simulink model "AXI_QPSK_Tx"  (R2023b)
settings: Solver=FixedStepAuto  StartTime=0.0  StopTime=10/Rb  RelTol=1e-3
PreLoadFcn:
  | Rb = 1000;   % 1kbit / s
  | Rsym = Rb/2;   % 2 bits per symbol
  | Rsymbol = Rb/2;
  | OSR = 32;
  | f_error = 120;
  | 
  | design_filters_tx
values from neighbouring files (symbols this model uses):
  CIC_fine_Tx = 2^-(CIC_right_shift - CIC_left_shift - CIC_shift_Tx)    [design_filters_tx.m]
  fCIC = fCICcomp * R_CIC    (= 25600000)    [design_filters_tx.m]
  fHB = fRRC * R_HB    (= 4000)    [design_filters_tx.m]
  R_CICcomp = 2    [design_filters_tx.m]
  R_HB = 2    [design_filters_tx.m]
  R_RRC = 4    [design_filters_tx.m]
undefined symbols (not defined in the file or in its folder): AXI4, Lite
libraries: hdlBasic x309, hdlDSPIP x8, hdlsllib x2, vmcUtilities x1
(part 2 of 4)

== system AXI_QPSK_Tx/AXI_QPSK_Generator/M_AXIS_FFT ==
  tdata_in : Inport
  tvalid_in : Inport  Port=2
  tlast_in : Inport  Port=3
  tready_in : Inport  Port=4
  m_fft_axis_tdata : hdlBasic/Gateway Out  inherit_from_input=on  hdl_port=on  rows=1  columns=1  UseAsDAC=off  DACChannel='1'  interface=None  automatic_assignment=on  address_offset=hex2dec('00')  intf_name=''  intf_description=''  timing_constraint=None  locs_specified=off  LOCs={}  io_standard={}  XmcBlockStatus=1  maskContainerNames=group4  block_type=gatewayout  block_config=sysgen:gateway_out_config  block_width_w=590  block_height_w=620  block_width=620  block_height=750
  m_fft_axis_tlast : hdlBasic/Gateway Out  inherit_from_input=off  hdl_port=on  rows=1  columns=1  UseAsDAC=off  DACChannel='1'  interface=None  automatic_assignment=on  address_offset=hex2dec('00')  intf_name=''  intf_description=''  timing_constraint=None  locs_specified=off  LOCs={}  io_standard={}  XmcBlockStatus=1  maskContainerNames=group4  block_type=gatewayout  block_config=sysgen:gateway_out_config  block_width_w=590  block_height_w=620  block_width=620  block_height=750
  m_fft_axis_tready : hdlBasic/Gateway In  gui_display_data_type=Boolean  arith_type=Boolean  n_bits=16  bin_pt=14  preci_type=Single  exp_width=8  frac_width=24  rows=1  columns=1  quantization="Round  (unbiased: +/- Inf)"  overflow=Saturate  period=1/(fCIC)  UseAsADC=off  ADCChannel='1'  interface=None  automatic_assignment=on  address_offset=hex2dec('00')  intf_name=''  intf_description=''  default_value=0  timing_constraint=None  locs_specified=off  LOCs={}  io_standard={}  inherit_from_input=off  hdl_port=on  XmcBlockStatus=1  maskContainerNames=group4  block_type=gatewayin  block_config=sysgen:gateway_in_config  block_width_w=590  block_height_w=620  block_width=640  block_height=850
  m_fft_axis_tvalid : hdlBasic/Gateway Out  inherit_from_input=off  hdl_port=on  rows=1  columns=1  UseAsDAC=off  DACChannel='1'  interface=None  automatic_assignment=on  address_offset=hex2dec('00')  intf_name=''  intf_description=''  timing_constraint=None  locs_specified=off  LOCs={}  io_standard={}  XmcBlockStatus=1  maskContainerNames=group4  block_type=gatewayout  block_config=sysgen:gateway_out_config  block_width_w=590  block_height_w=620  block_width=620  block_height=750
  tdata_out : Outport  VectorParamsAs1DForOutWhenUnconnected=off
  tvalid_out : Outport  Port=2  VectorParamsAs1DForOutWhenUnconnected=off
  tlast_out : Outport  Port=3  VectorParamsAs1DForOutWhenUnconnected=off
  tready_out : Outport  Port=4  VectorParamsAs1DForOutWhenUnconnected=off
  wires:
  tready_in/1 -> m_fft_axis_tready/1
  m_fft_axis_tdata/1 -> tdata_out/1
  tdata_in/1 -> m_fft_axis_tdata/1
  m_fft_axis_tvalid/1 -> tvalid_out/1
  tvalid_in/1 -> m_fft_axis_tvalid/1
  m_fft_axis_tready/1 -> tready_out/1
  m_fft_axis_tlast/1 -> tlast_out/1
  tlast_in/1 -> m_fft_axis_tlast/1

== system AXI_QPSK_Tx/AXI_QPSK_Generator/M_AXIS_SYMBOL ==
  tdata_in : Inport
  tvalid_in : Inport  Port=2
  tlast_in : Inport  Port=3
  tready_in : Inport  Port=4
  m_symbol_axis_tdata : hdlBasic/Gateway Out  inherit_from_input=on  hdl_port=on  rows=1  columns=1  UseAsDAC=off  DACChannel='1'  interface=None  automatic_assignment=on  address_offset=hex2dec('00')  intf_name=''  intf_description=''  timing_constraint=None  locs_specified=off  LOCs={}  io_standard={}  XmcBlockStatus=1  maskContainerNames=group4  block_type=gatewayout  block_config=sysgen:gateway_out_config  block_width_w=590  block_height_w=620  block_width=620  block_height=750
  m_symbol_axis_tlast : hdlBasic/Gateway Out  inherit_from_input=off  hdl_port=on  rows=1  columns=1  UseAsDAC=off  DACChannel='1'  interface=None  automatic_assignment=on  address_offset=hex2dec('00')  intf_name=''  intf_description=''  timing_constraint=None  locs_specified=off  LOCs={}  io_standard={}  XmcBlockStatus=1  maskContainerNames=group4  block_type=gatewayout  block_config=sysgen:gateway_out_config  block_width_w=590  block_height_w=620  block_width=620  block_height=750
  m_symbol_axis_tready : hdlBasic/Gateway In  gui_display_data_type=Boolean  arith_type=Boolean  n_bits=16  bin_pt=14  preci_type=Single  exp_width=8  frac_width=24  rows=1  columns=1  quantization="Round  (unbiased: +/- Inf)"  overflow=Saturate  period=1/(fCIC)  UseAsADC=off  ADCChannel='1'  interface=None  automatic_assignment=on  address_offset=hex2dec('00')  intf_name=''  intf_description=''  default_value=0  timing_constraint=None  locs_specified=off  LOCs={}  io_standard={}  inherit_from_input=off  hdl_port=on  XmcBlockStatus=1  maskContainerNames=group4  block_type=gatewayin  block_config=sysgen:gateway_in_config  block_width_w=590  block_height_w=620  block_width=640  block_height=850
  m_symbol_axis_tvalid : hdlBasic/Gateway Out  inherit_from_input=off  hdl_port=on  rows=1  columns=1  UseAsDAC=off  DACChannel='1'  interface=None  automatic_assignment=on  address_offset=hex2dec('00')  intf_name=''  intf_description=''  timing_constraint=None  locs_specified=off  LOCs={}  io_standard={}  XmcBlockStatus=1  maskContainerNames=group4  block_type=gatewayout  block_config=sysgen:gateway_out_config  block_width_w=590  block_height_w=620  block_width=620  block_height=750
  tdata_out : Outport  VectorParamsAs1DForOutWhenUnconnected=off
  tvalid_out : Outport  Port=2  VectorParamsAs1DForOutWhenUnconnected=off
  tlast_out : Outport  Port=3  VectorParamsAs1DForOutWhenUnconnected=off
  tready_out : Outport  Port=4  VectorParamsAs1DForOutWhenUnconnected=off
  wires:
  tlast_in/1 -> m_symbol_axis_tlast/1
  m_symbol_axis_tlast/1 -> tlast_out/1
  m_symbol_axis_tready/1 -> tready_out/1
  tvalid_in/1 -> m_symbol_axis_tvalid/1
  m_symbol_axis_tvalid/1 -> tvalid_out/1
  tdata_in/1 -> m_symbol_axis_tdata/1
  m_symbol_axis_tdata/1 -> tdata_out/1
  tready_in/1 -> m_symbol_axis_tready/1

== system AXI_QPSK_Tx/AXI_QPSK_Generator/M_AXIS_TIME ==
  tdata_in : Inport
  tvalid_in : Inport  Port=2
  tlast_in : Inport  Port=3
  tready_in : Inport  Port=4
  m_time_axis_tdata : hdlBasic/Gateway Out  inherit_from_input=on  hdl_port=on  rows=1  columns=1  UseAsDAC=off  DACChannel='1'  interface=None  automatic_assignment=on  address_offset=hex2dec('00')  intf_name=''  intf_description=''  timing_constraint=None  locs_specified=off  LOCs={}  io_standard={}  XmcBlockStatus=1  maskContainerNames=group4  block_type=gatewayout  block_config=sysgen:gateway_out_config  block_width_w=590  block_height_w=620  block_width=620  block_height=750
  m_time_axis_tlast : hdlBasic/Gateway Out  inherit_from_input=off  hdl_port=on  rows=1  columns=1  UseAsDAC=off  DACChannel='1'  interface=None  automatic_assignment=on  address_offset=hex2dec('00')  intf_name=''  intf_description=''  timing_constraint=None  locs_specified=off  LOCs={}  io_standard={}  XmcBlockStatus=1  maskContainerNames=group4  block_type=gatewayout  block_config=sysgen:gateway_out_config  block_width_w=590  block_height_w=620  block_width=620  block_height=750
  m_time_axis_tready : hdlBasic/Gateway In  gui_display_data_type=Boolean  arith_type=Boolean  n_bits=16  bin_pt=14  preci_type=Single  exp_width=8  frac_width=24  rows=1  columns=1  quantization="Round  (unbiased: +/- Inf)"  overflow=Saturate  period=1/(fCIC)  UseAsADC=off  ADCChannel='1'  interface=None  automatic_assignment=on  address_offset=hex2dec('00')  intf_name=''  intf_description=''  default_value=0  timing_constraint=None  locs_specified=off  LOCs={}  io_standard={}  inherit_from_input=off  hdl_port=on  XmcBlockStatus=1  maskContainerNames=group4  block_type=gatewayin  block_config=sysgen:gateway_in_config  block_width_w=590  block_height_w=620  block_width=640  block_height=850
  m_time_axis_tvalid : hdlBasic/Gateway Out  inherit_from_input=off  hdl_port=on  rows=1  columns=1  UseAsDAC=off  DACChannel='1'  interface=None  automatic_assignment=on  address_offset=hex2dec('00')  intf_name=''  intf_description=''  timing_constraint=None  locs_specified=off  LOCs={}  io_standard={}  XmcBlockStatus=1  maskContainerNames=group4  block_type=gatewayout  block_config=sysgen:gateway_out_config  block_width_w=590  block_height_w=620  block_width=620  block_height=750
  tdata_out : Outport  VectorParamsAs1DForOutWhenUnconnected=off
  tvalid_out : Outport  Port=2  VectorParamsAs1DForOutWhenUnconnected=off
  tlast_out : Outport  Port=3  VectorParamsAs1DForOutWhenUnconnected=off
  tready_out : Outport  Port=4  VectorParamsAs1DForOutWhenUnconnected=off
  wires:
  tready_in/1 -> m_time_axis_tready/1
  m_time_axis_tdata/1 -> tdata_out/1
  tdata_in/1 -> m_time_axis_tdata/1
  m_time_axis_tvalid/1 -> tvalid_out/1
  tvalid_in/1 -> m_time_axis_tvalid/1
  m_time_axis_tready/1 -> tready_out/1
  m_time_axis_tlast/1 -> tlast_out/1
  tlast_in/1 -> m_time_axis_tlast/1

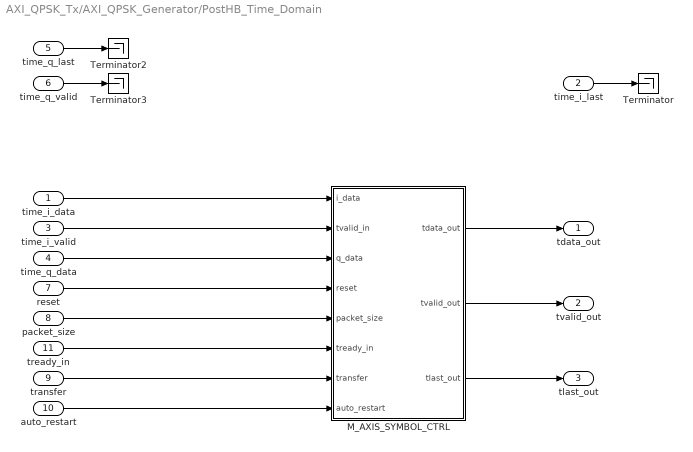
== system AXI_QPSK_Tx/AXI_QPSK_Generator/PostHB_Time_Domain ==
  time_i_data : Inport
  time_i_last : Inport  Port=2
  time_i_valid : Inport  Port=3
  time_q_data : Inport  Port=4
  time_q_last : Inport  Port=5
  time_q_valid : Inport  Port=6
  reset : Inport  Port=7
  packet_size : Inport  Port=8
  transfer : Inport  Port=9
  auto_restart : Inport  Port=10
  tready_in : Inport  Port=11
  M_AXIS_SYMBOL_CTRL : Subsystem
  Terminator : Terminator
  Terminator2 : Terminator
  Terminator3 : Terminator
  tdata_out : Outport  VectorParamsAs1DForOutWhenUnconnected=off
  tvalid_out : Outport  Port=2  VectorParamsAs1DForOutWhenUnconnected=off
  tlast_out : Outport  Port=3  VectorParamsAs1DForOutWhenUnconnected=off
  wires:
  auto_restart/1 -> M_AXIS_SYMBOL_CTRL/8(auto_restart)
  transfer/1 -> M_AXIS_SYMBOL_CTRL/7(transfer)
  M_AXIS_SYMBOL_CTRL/3(tlast_out) -> tlast_out/1
  M_AXIS_SYMBOL_CTRL/2(tvalid_out) -> tvalid_out/1
  M_AXIS_SYMBOL_CTRL/1(tdata_out) -> tdata_out/1
  tready_in/1 -> M_AXIS_SYMBOL_CTRL/6(tready_in)
  packet_size/1 -> M_AXIS_SYMBOL_CTRL/5(packet_size)
  reset/1 -> M_AXIS_SYMBOL_CTRL/4(reset)
  time_q_data/1 -> M_AXIS_SYMBOL_CTRL/3(q_data)
  time_i_valid/1 -> M_AXIS_SYMBOL_CTRL/2(tvalid_in)
  time_i_data/1 -> M_AXIS_SYMBOL_CTRL/1(i_data)
  time_q_valid/1 -> Terminator3/1
  time_q_last/1 -> Terminator2/1
  time_i_last/1 -> Terminator/1

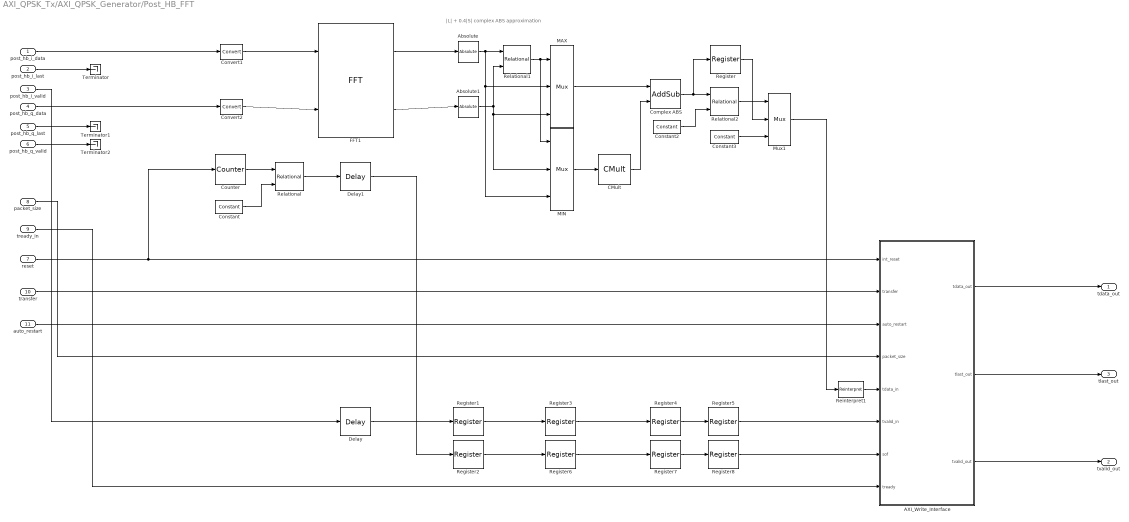
== system AXI_QPSK_Tx/AXI_QPSK_Generator/Post_HB_FFT ==
  note: |L| + 0.4|S| complex ABS approximation
  post_hb_i_data : Inport
  post_hb_i_last : Inport  Port=2
  post_hb_i_valid : Inport  Port=3
  post_hb_q_data : Inport  Port=4
  post_hb_q_last : Inport  Port=5
  post_hb_q_valid : Inport  Port=6
  reset : Inport  Port=7
  packet_size : Inport  Port=8
  tready_in : Inport  Port=9
  transfer : Inport  Port=10
  auto_restart : Inport  Port=11
  AXI_Write_Interface : Subsystem
  Absolute : hdlBasic/Absolute  precision=User Defined  arith_type=Unsigned  n_bits=32  bin_pt=31  quantization=Truncate  overflow=Wrap  en=off  latency=1  XmcBlockStatus=1  maskContainerNames=tabcontainer1  block_type=abs  block_config=sysgen:Abs_config
  Absolute1 : hdlBasic/Absolute  precision=User Defined  arith_type=Unsigned  n_bits=32  bin_pt=31  quantization=Truncate  overflow=Wrap  en=off  latency=1  XmcBlockStatus=1  maskContainerNames=tabcontainer1  block_type=abs  block_config=sysgen:Abs_config
  CMult : hdlBasic/CMult  const=0.4  gui_display_data_type=Fixed-point  const_n_bits=32  const_bin_pt=31  float_type=Single  exp_bits=8  fraction_bits=24  en=off  latency=0  precision=Full  arith_type=Unsigned  n_bits=15  bin_pt=15  quantization=Truncate  overflow=Wrap  use_behavioral_HDL=off  mem_type=Distributed RAM  pipeline=off  XmcBlockStatus=1  maskContainerNames=tabcontainer1  block_type=cmult  block_config=sysgen:CMult_config
      settings: infoedit=[]
  Complex ABS : hdlBasic/AddSub  mode=Addition  use_carryin=off  use_carryout=off  en=off  latency=1  precision=User Defined  arith_type=Unsigned  n_bits=32  bin_pt=31  quantization=Truncate  overflow=Wrap  use_behavioral_HDL=off  hw_selection=Fabric  pipelined=off  XmcBlockStatus=1  maskContainerNames=tabcontainer1  block_type=addsub  block_config=sysgen:Addsub_config
  Constant : hdlBasic/Constant  const=0  gui_display_data_type=Fixed-point  arith_type=Unsigned  n_bits=10  bin_pt=0  preci_type=Single  exp_width=8  frac_width=24  explicit_period=on  period=1/fHB  XmcBlockStatus=1  maskContainerNames=tabcontainer1  block_type=constant  block_config=sysgen:Constant_config
  Constant2 : hdlBasic/Constant  const=0  gui_display_data_type=Fixed-point  arith_type=Unsigned  n_bits=32  bin_pt=31  preci_type=Single  exp_width=8  frac_width=24  explicit_period=on  period=1/fHB  XmcBlockStatus=1  maskContainerNames=tabcontainer1  block_type=constant  block_config=sysgen:Constant_config
  Constant3 : hdlBasic/Constant  const=2^-31  gui_display_data_type=Fixed-point  arith_type=Unsigned  n_bits=32  bin_pt=31  preci_type=Single  exp_width=8  frac_width=24  explicit_period=on  period=1/fHB  XmcBlockStatus=1  maskContainerNames=tabcontainer1  block_type=constant  block_config=sysgen:Constant_config
  Convert1 : hdlBasic/Convert  gui_display_data_type=Fixed-point  arith_type="Signed  (2's comp)"  n_bits=32  bin_pt=31  float_type=Single  exp_bits=8  fraction_bits=24  quantization=Truncate  overflow=Wrap  en=off  latency=0  pipeline=off  XmcBlockStatus=1  maskContainerNames=group2  block_type=convert  block_config=sysgen:Convert_config  block_width=595  block_height=885
  Convert2 : hdlBasic/Convert  gui_display_data_type=Fixed-point  arith_type="Signed  (2's comp)"  n_bits=32  bin_pt=31  float_type=Single  exp_bits=8  fraction_bits=24  quantization=Truncate  overflow=Wrap  en=off  latency=0  pipeline=off  XmcBlockStatus=1  maskContainerNames=group2  block_type=convert  block_config=sysgen:Convert_config  block_width=595  block_height=885
  Counter : hdlBasic/Counter  cnt_type=Count limited  cnt_to=1023  operation=Up  start_count=0  cnt_by_val=1  arith_type=Unsigned  n_bits=10  bin_pt=0  load_pin=off  rst=on  en=off  explicit_period=Explicit  period=1/fHB  use_behavioral_HDL=off  implementation=Fabric  XmcBlockStatus=1  maskContainerNames=group1  block_type=counter  block_config=sysgen:Counter_config  block_width=531  block_height=1023
  Delay : hdlBasic/Delay  rst=off  en=off  latency=2204  reg_retiming=off  XmcBlockStatus=1  maskContainerNames=group1  block_type=delay  block_config=sysgen:Delay_config
  Delay1 : hdlBasic/Delay  rst=off  en=off  latency=2204  reg_retiming=off  XmcBlockStatus=1  maskContainerNames=group1  block_type=delay  block_config=sysgen:Delay_config
  FFT1 : hdlBasic/FFT  transform_length=1024  scale_result_by_fft_length=on  bit_reversed_order=on  optimizegoal=Performance  start_frame=off  simulation_type=fast_sim  simulation_model=sysgen:ForwardFFT_Macro  latency=1  XmcBlockStatus=1  maskContainerNames=group1  block_type=xfft_forward  block_config=sysgen:FFTMacro_config
  MAX : hdlBasic/Mux  inputs=2  en=off  latency=1  precision=Full  arith_type=Unsigned  n_bits=16  bin_pt=14  quantization=Truncate  overflow=Wrap  XmcBlockStatus=1  maskContainerNames=tabcontainer1  block_type=mux  block_config=sysgen:Mux_config
  MIN : hdlBasic/Mux  inputs=2  en=off  latency=1  precision=Full  arith_type=Unsigned  n_bits=16  bin_pt=14  quantization=Truncate  overflow=Wrap  XmcBlockStatus=1  maskContainerNames=tabcontainer1  block_type=mux  block_config=sysgen:Mux_config
  Mux1 : hdlBasic/Mux  inputs=2  en=off  latency=0  precision=Full  arith_type=Unsigned  n_bits=16  bin_pt=14  quantization=Truncate  overflow=Wrap  XmcBlockStatus=1  maskContainerNames=tabcontainer1  block_type=mux  block_config=sysgen:Mux_config
  Register{,1..8} (9 alike) : hdlBasic/Register  init=0  rst=off  en=off  XmcBlockStatus=1  maskContainerNames=tabcontainer1  block_type=register  block_config=sysgen:Register_config
  Reinterpret1 : hdlBasic/Reinterpret  force_arith_type=on  arith_type=Unsigned  force_bin_pt=on  bin_pt=0  XmcBlockStatus=1  maskContainerNames=group1  block_type=reinterpret  block_config=sysgen:Reinterpret_config
  Relational : hdlBasic/Relational  mode=a=b  op_type=Bool  en=off  latency=0  XmcBlockStatus=1  maskContainerNames=tabcontainer1  block_type=relational  block_config=sysgen:Relational_config
  Relational1 : hdlBasic/Relational  mode=a<b  op_type=Bool  en=off  latency=0  XmcBlockStatus=1  maskContainerNames=tabcontainer1  block_type=relational  block_config=sysgen:Relational_config
  Relational2 : hdlBasic/Relational  mode=a=b  op_type=Bool  en=off  latency=1  XmcBlockStatus=1  maskContainerNames=tabcontainer1  block_type=relational  block_config=sysgen:Relational_config
  Terminator : Terminator
  Terminator1 : Terminator
  Terminator2 : Terminator
  tdata_out : Outport  VectorParamsAs1DForOutWhenUnconnected=off
  tvalid_out : Outport  Port=2  VectorParamsAs1DForOutWhenUnconnected=off
  tlast_out : Outport  Port=3  VectorParamsAs1DForOutWhenUnconnected=off
  wires:
  post_hb_i_last/1 -> Terminator/1
  post_hb_q_last/1 -> Terminator1/1
  post_hb_q_valid/1 -> Terminator2/1
  AXI_Write_Interface/3(tvalid_out) -> tvalid_out/1
  AXI_Write_Interface/2(tlast_out) -> tlast_out/1
  packet_size/1 -> AXI_Write_Interface/4(packet_size)
  post_hb_i_valid/1 -> Delay/1
  Delay/1 -> Register1/1
  reset/1 -> Counter/1, AXI_Write_Interface/1(int_reset)
  FFT1/1 -> Absolute/1
  Relational1/1 -> MAX/1, MIN/1
  CMult/1 -> Complex ABS/2
  MAX/1 -> Complex ABS/1
  MIN/1 -> CMult/1
  Absolute1/1 -> MIN/2, MAX/3, Relational1/2
  Absolute/1 -> MAX/2, MIN/3, Relational1/1
  FFT1/2 -> Absolute1/1
  post_hb_i_data/1 -> Convert1/1
  AXI_Write_Interface/1(tdata_out) -> tdata_out/1
  transfer/1 -> AXI_Write_Interface/2(transfer)
  auto_restart/1 -> AXI_Write_Interface/3(auto_restart)
  Relational/1 -> Delay1/1
  tready_in/1 -> AXI_Write_Interface/8(tready)
  post_hb_q_data/1 -> Convert2/1
  Convert1/1 -> FFT1/1
  Convert2/1 -> FFT1/2
  Complex ABS/1 -> Register/1, Relational2/1
  Constant2/1 -> Relational2/2
  Relational2/1 -> Mux1/1
  Constant3/1 -> Mux1/3
  Register/1 -> Mux1/2
  Mux1/1 -> Reinterpret1/1
  Reinterpret1/1 -> AXI_Write_Interface/5(tdata_in)
  Counter/1 -> Relational/1
  Constant/1 -> Relational/2
  Delay1/1 -> Register2/1
  Register1/1 -> Register3/1
  Register2/1 -> Register6/1
  Register3/1 -> Register4/1
  Register4/1 -> Register5/1
  Register5/1 -> AXI_Write_Interface/6(tvalid_in)
  Register6/1 -> Register7/1
  Register7/1 -> Register8/1
  Register8/1 -> AXI_Write_Interface/7(sof)

== system AXI_QPSK_Tx/AXI_QPSK_Generator/QPSK_symbol_mapper ==
  note: Symbol rate =
      | 500sps
  Bit_pairs : Inport
  tlast_in : Inport  Port=2
  Reset : Inport  Port=3
  tready : Inport  Port=4
  Constant : hdlBasic/Constant  const=1.0  gui_display_data_type=Fixed-point  arith_type=Signed (2's comp)  n_bits=2  bin_pt=0  preci_type=Single  exp_width=8  frac_width=24  explicit_period=on  period=2/Rb  XmcBlockStatus=1  maskContainerNames=tabcontainer1  block_type=constant  block_config=sysgen:Constant_config
  Constant1 : hdlBasic/Constant  const=-1  gui_display_data_type=Fixed-point  arith_type=Signed (2's comp)  n_bits=2  bin_pt=0  preci_type=Single  exp_width=8  frac_width=24  explicit_period=on  period=2/Rb  XmcBlockStatus=1  maskContainerNames=tabcontainer1  block_type=constant  block_config=sysgen:Constant_config
  Constant2 : hdlBasic/Constant  const=1.0  gui_display_data_type=Fixed-point  arith_type=Signed (2's comp)  n_bits=2  bin_pt=0  preci_type=Single  exp_width=8  frac_width=24  explicit_period=on  period=2/Rb  XmcBlockStatus=1  maskContainerNames=tabcontainer1  block_type=constant  block_config=sysgen:Constant_config
  Constant3 : hdlBasic/Constant  const=-1  gui_display_data_type=Fixed-point  arith_type=Signed (2's comp)  n_bits=2  bin_pt=0  preci_type=Single  exp_width=8  frac_width=24  explicit_period=on  period=2/Rb  XmcBlockStatus=1  maskContainerNames=tabcontainer1  block_type=constant  block_config=sysgen:Constant_config
  Mux : hdlBasic/Mux  inputs=4  en=off  latency=0  precision=User Defined  arith_type="Signed  (2's comp)"  n_bits=2  bin_pt=0  quantization=Truncate  overflow=Wrap  XmcBlockStatus=1  maskContainerNames=tabcontainer1  block_type=mux  block_config=sysgen:Mux_config
  Mux1 : hdlBasic/Mux  inputs=4  en=off  latency=0  precision=User Defined  arith_type="Signed  (2's comp)"  n_bits=2  bin_pt=0  quantization=Truncate  overflow=Wrap  XmcBlockStatus=1  maskContainerNames=tabcontainer1  block_type=mux  block_config=sysgen:Mux_config
  Register : hdlBasic/Register  init=0  rst=on  en=on  XmcBlockStatus=1  maskContainerNames=tabcontainer1  block_type=register  block_config=sysgen:Register_config
  Register1 : hdlBasic/Register  init=0  rst=on  en=on  XmcBlockStatus=1  maskContainerNames=tabcontainer1  block_type=register  block_config=sysgen:Register_config
  Register2 : hdlBasic/Register  init=0  rst=on  en=on  XmcBlockStatus=1  maskContainerNames=tabcontainer1  block_type=register  block_config=sysgen:Register_config
  I_symbols : Outport  VectorParamsAs1DForOutWhenUnconnected=off
  Q_symbols : Outport  Port=2  VectorParamsAs1DForOutWhenUnconnected=off
  tlast_out : Outport  Port=3  VectorParamsAs1DForOutWhenUnconnected=off
  wires:
  Constant/1 -> Mux/3, Mux/2
  Constant3/1 -> Mux1/3, Mux1/5
  Register/1 -> I_symbols/1
  Bit_pairs/1 -> Mux/1, Mux1/1
  Constant2/1 -> Mux1/4, Mux1/2
  Mux/1 -> Register/1
  Mux1/1 -> Register1/1
  Constant1/1 -> Mux/5, Mux/4
  Register1/1 -> Q_symbols/1
  Reset/1 -> Register2/2, Register/2, Register1/2
  tready/1 -> Register/3, Register1/3, Register2/3
  tlast_in/1 -> Register2/1
  Register2/1 -> tlast_out/1

== system AXI_QPSK_Tx/AXI_QPSK_Generator/RF_Output ==
  rf_i_data : Inport
  rf_i_valid : Inport  Port=2
  rf_i_last : Inport  Port=3
  rf_q_data : Inport  Port=4
  rf_q_valid : Inport  Port=5
  rf_q_last : Inport  Port=6
  rf_ch_sel : Inport  Port=7
  Concat : hdlBasic/Concat  num_inputs=2  XmcBlockStatus=1  maskContainerNames=group1  block_type=concat  block_config=sysgen:Concat_config
  Logical1 : hdlBasic/Logical  logical_function=AND  inputs=2  en=off  latency=0  precision=Full  arith_type=Unsigned  n_bits=16  bin_pt=0  align_bp=on  overflow=[]  quantization=[]  XmcBlockStatus=1  maskContainerNames=tabcontainer1  block_type=logical  block_config=sysgen:Logical_config
  Logical2 : hdlBasic/Logical  logical_function=AND  inputs=2  en=off  latency=0  precision=Full  arith_type=Unsigned  n_bits=16  bin_pt=0  align_bp=on  overflow=[]  quantization=[]  XmcBlockStatus=1  maskContainerNames=tabcontainer1  block_type=logical  block_config=sysgen:Logical_config
  channel_selector : Subsystem
  ch0_out : Outport  VectorParamsAs1DForOutWhenUnconnected=off
  tvalid_in : Outport  Port=2  VectorParamsAs1DForOutWhenUnconnected=off
  tlast_in : Outport  Port=3  VectorParamsAs1DForOutWhenUnconnected=off
  ch1_out : Outport  Port=4  VectorParamsAs1DForOutWhenUnconnected=off
  ch2_out : Outport  Port=5  VectorParamsAs1DForOutWhenUnconnected=off
  ch3_out : Outport  Port=6  VectorParamsAs1DForOutWhenUnconnected=off
  wires:
  rf_q_data/1 -> Concat/1
  rf_i_last/1 -> Logical2/1
  rf_q_valid/1 -> Logical1/2
  rf_i_valid/1 -> Logical1/1
  Logical2/1 -> tlast_in/1
  rf_q_last/1 -> Logical2/2
  Logical1/1 -> tvalid_in/1
  rf_i_data/1 -> Concat/2
  channel_selector/1(ch0_out) -> ch0_out/1
  channel_selector/2(ch1_out) -> ch1_out/1
  channel_selector/3(ch2_out) -> ch2_out/1
  channel_selector/4(ch3_out) -> ch3_out/1
  Concat/1 -> channel_selector/2(data_in)
  rf_ch_sel/1 -> channel_selector/1(ch_sel)

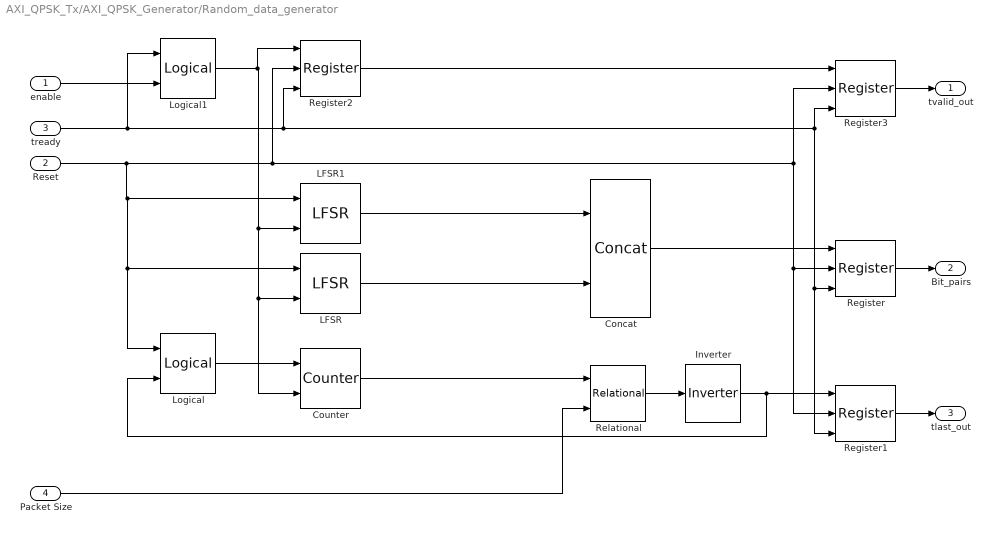
== system AXI_QPSK_Tx/AXI_QPSK_Generator/Random_data_generator ==
  enable : Inport
  Reset : Inport  Port=2
  tready : Inport  Port=3
  Packet Size : Inport  Port=4
  Concat : hdlBasic/Concat  num_inputs=2  XmcBlockStatus=1  maskContainerNames=group1  block_type=concat  block_config=sysgen:Concat_config
  Counter : hdlBasic/Counter  cnt_type=Free running  cnt_to=Inf  operation=Up  start_count=0  cnt_by_val=1  arith_type=Unsigned  n_bits=32  bin_pt=0  load_pin=off  rst=on  en=on  explicit_period=Explicit  period=2/Rb  use_behavioral_HDL=off  implementation=Fabric  XmcBlockStatus=1  maskContainerNames=group1  block_type=counter  block_config=sysgen:Counter_config  block_width=531  block_height=1023
  Inverter : hdlBasic/Inverter  en=off  latency=0  XmcBlockStatus=1  maskContainerNames=group2  block_type=inv  block_config=sysgen:Inverter_config
  LFSR : hdlBasic/LFSR  lfsr_type=Fibonacci  gate_type=XNOR  n_bits=10  maxpolynomial=on  polynomial='121'  rst_value='011'  rst=on  en=on  reloadable_seed=off  input_type=off  output_type=off  arith_type="Signed  (2's comp)"  bin_pt=4  explicit_period=on  period=2/Rb  XmcBlockStatus=1  maskContainerNames=tabcontainer1  block_type=lfsr  block_config=sysgen:LFSR_config
  LFSR1 : hdlBasic/LFSR  lfsr_type=Fibonacci  gate_type=XNOR  n_bits=10  maxpolynomial=on  polynomial='121'  rst_value='001'  rst=on  en=on  reloadable_seed=off  input_type=off  output_type=off  arith_type="Signed  (2's comp)"  bin_pt=4  explicit_period=on  period=2/Rb  XmcBlockStatus=1  maskContainerNames=tabcontainer1  block_type=lfsr  block_config=sysgen:LFSR_config
  Logical : hdlBasic/Logical  logical_function=OR  inputs=2  en=off  latency=0  precision=Full  arith_type=Unsigned  n_bits=16  bin_pt=0  align_bp=on  overflow=[]  quantization=[]  XmcBlockStatus=1  maskContainerNames=tabcontainer1  block_type=logical  block_config=sysgen:Logical_config
  Logical1 : hdlBasic/Logical  logical_function=AND  inputs=2  en=off  latency=0  precision=Full  arith_type=Unsigned  n_bits=16  bin_pt=0  align_bp=on  overflow=[]  quantization=[]  XmcBlockStatus=1  maskContainerNames=tabcontainer1  block_type=logical  block_config=sysgen:Logical_config
  Register{,1..3} (4 alike) : hdlBasic/Register  init=0  rst=on  en=on  XmcBlockStatus=1  maskContainerNames=tabcontainer1  block_type=register  block_config=sysgen:Register_config
  Relational : hdlBasic/Relational  mode=a<b  op_type=Bool  en=off  latency=0  XmcBlockStatus=1  maskContainerNames=tabcontainer1  block_type=relational  block_config=sysgen:Relational_config
  tvalid_out : Outport  VectorParamsAs1DForOutWhenUnconnected=off
  Bit_pairs : Outport  Port=2  VectorParamsAs1DForOutWhenUnconnected=off
  tlast_out : Outport  Port=3  VectorParamsAs1DForOutWhenUnconnected=off
  wires:
  tready/1 -> Logical1/1, Register1/3, Register/3, Register3/3, Register2/3
  Logical/1 -> Counter/1
  Concat/1 -> Register/1
  Register/1 -> Bit_pairs/1
  Reset/1 -> LFSR1/1, LFSR/1, Logical/1, Register3/2, Register1/2, Register/2, Register2/2
  Register1/1 -> tlast_out/1
  Relational/1 -> Inverter/1
  Inverter/1 -> Logical/2, Register1/1
  Packet Size/1 -> Relational/2
  enable/1 -> Logical1/2
  Logical1/1 -> Register2/1, LFSR1/2, LFSR/2, Counter/2
  Register3/1 -> tvalid_out/1
  LFSR/1 -> Concat/2
  LFSR1/1 -> Concat/1
  Counter/1 -> Relational/1
  Register2/1 -> Register3/1

== system AXI_QPSK_Tx/AXI_QPSK_Generator/Symbol_2_Output ==
  symbol_i_data : Inport
  symbol_i_last : Inport  Port=2
  symbol_i_valid : Inport  Port=3
  symbol_q_data : Inport  Port=4
  symbol_q_last : Inport  Port=5
  symbol_q_valid : Inport  Port=6
  reset : Inport  Port=7
  packet_size : Inport  Port=8
  transfer : Inport  Port=9
  auto_restart : Inport  Port=10
  tready_in : Inport  Port=11
  M_AXIS_SYMBOL_CTRL : Subsystem
  Terminator : Terminator
  Terminator2 : Terminator
  Terminator3 : Terminator
  tdata_out : Outport  VectorParamsAs1DForOutWhenUnconnected=off
  tvalid_out : Outport  Port=2  VectorParamsAs1DForOutWhenUnconnected=off
  tlast_out : Outport  Port=3  VectorParamsAs1DForOutWhenUnconnected=off
  wires:
  symbol_i_last/1 -> Terminator/1
  symbol_q_last/1 -> Terminator2/1
  symbol_q_valid/1 -> Terminator3/1
  symbol_i_data/1 -> M_AXIS_SYMBOL_CTRL/1(i_data)
  symbol_i_valid/1 -> M_AXIS_SYMBOL_CTRL/2(tvalid_in)
  symbol_q_data/1 -> M_AXIS_SYMBOL_CTRL/3(q_data)
  reset/1 -> M_AXIS_SYMBOL_CTRL/4(reset)
  packet_size/1 -> M_AXIS_SYMBOL_CTRL/5(packet_size)
  tready_in/1 -> M_AXIS_SYMBOL_CTRL/6(tready_in)
  M_AXIS_SYMBOL_CTRL/1(tdata_out) -> tdata_out/1
  M_AXIS_SYMBOL_CTRL/2(tvalid_out) -> tvalid_out/1
  M_AXIS_SYMBOL_CTRL/3(tlast_out) -> tlast_out/1
  transfer/1 -> M_AXIS_SYMBOL_CTRL/7(transfer)
  auto_restart/1 -> M_AXIS_SYMBOL_CTRL/8(auto_restart)
